simulink model "mainSIM"  (R2016a)
settings: Solver=VariableStepAuto  StartTime=0.0  StopTime=15  RelTol=1e-5
settings Model: Creator=Zoltan  LastModifiedBy=Zoltan

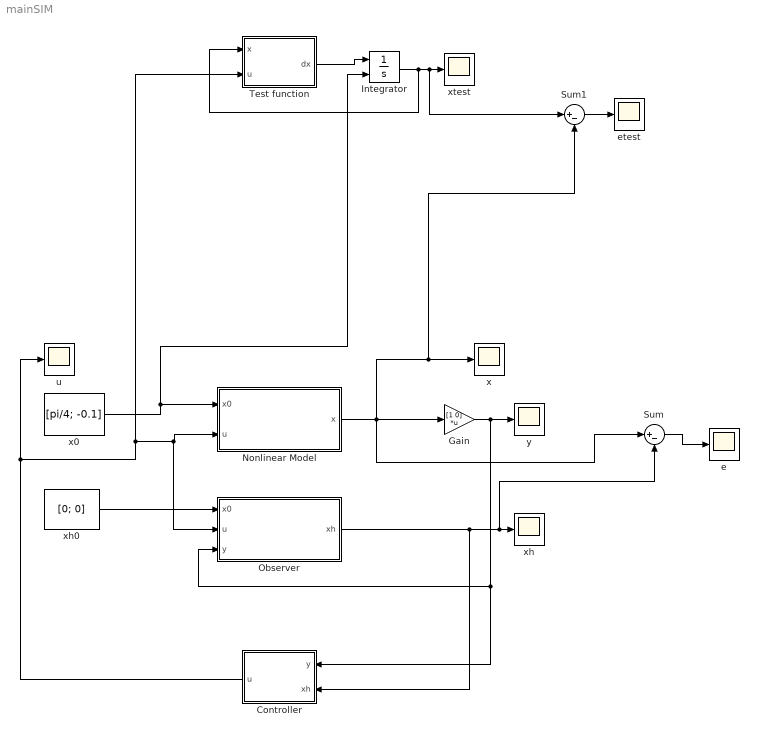
== system mainSIM ==
  Controller : MATLAB Function  TreatAsAtomicUnit=on
  Gain : Gain  Gain=[1 0]  Multiplication=Matrix(K*u) (u vector)
  Integrator : Integrator  InitialConditionSource=external
  Nonlinear Model : Subsystem
  Observer : Subsystem
  Sum : Sum  Inputs=|+-
  Sum1 : Sum  Inputs=|+-
  Test function : MATLAB Function  TreatAsAtomicUnit=on
  e : Scope
  etest : Scope
  "u " : Scope
  x : Scope
  x0 : Constant  Value=[pi/4; -0.1]
  xh : Scope
  xh0 : Constant  Value=[0; 0]
  xtest : Scope
  y : Scope
  wires:
  x0/1 -> Integrator/2, Nonlinear Model/1(x0)
  Controller/1(u) -> Test function/2(u), Observer/2(u), Nonlinear Model/2(u), "u "/1
  Nonlinear Model/1(x) -> Sum1/2, x/1, Sum/1, Gain/1
  Gain/1 -> Controller/1(y), Observer/3(y), y/1
  xh0/1 -> Observer/1(x0)
  Observer/1(xh) -> Controller/2(xh), Sum/2, xh/1
  Sum/1 -> e/1
  Test function/1(dx) -> Integrator/1
  Integrator/1 -> Test function/1(x), Sum1/1, xtest/1
  Sum1/1 -> etest/1

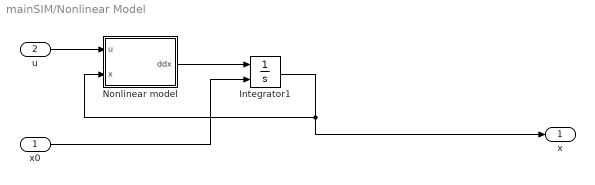
== system mainSIM/Nonlinear Model ==
  x0 : Inport
  u : Inport  Port=2
  Integrator1 : Integrator  InitialConditionSource=external
  Nonlinear model : MATLAB Function  TreatAsAtomicUnit=on
  x : Outport
  wires:
  u/1 -> Nonlinear model/1(u)
  x0/1 -> Integrator1/2
  Nonlinear model/1(ddx) -> Integrator1/1
  Integrator1/1 -> x/1, Nonlinear model/2(x)

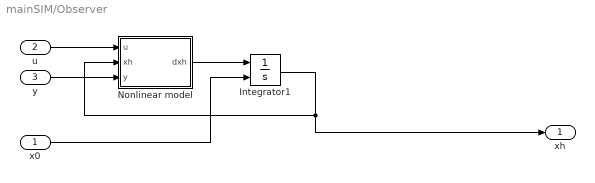
== system mainSIM/Observer ==
  x0 : Inport
  u : Inport  Port=2
  y : Inport  Port=3
  Integrator1 : Integrator  InitialConditionSource=external
  Nonlinear model : MATLAB Function  TreatAsAtomicUnit=on
  xh : Outport
  wires:
  u/1 -> Nonlinear model/1(u)
  x0/1 -> Integrator1/2
  Nonlinear model/1(dxh) -> Integrator1/1
  Integrator1/1 -> xh/1, Nonlinear model/2(xh)
  y/1 -> Nonlinear model/3(y)

== matlab function mainSIM/Observer/Nonlinear model ==
  data: u input; dxh output; xh input; y input
function dxh = fcn(u,xh,y)
coder.extrinsic('mydxh');
dxh= [0;0];
dxh = mydxh(y,xh,u);
y = u;

== matlab function mainSIM/Nonlinear Model/Nonlinear model ==
  data: u input; ddx output; x input
function ddx = fcn(u,x)
coder.extrinsic('mydx');
ddx= [0;0];
ddx = mydx(x,u);
y = u;

== matlab function mainSIM/Controller ==
  data: y input; xh input; u output
function u = fcn(y, xh)
coder.extrinsic('mycont');
u = 0;
u = mycont(y,xh);
%u = -u;
y = u;

== matlab function mainSIM/Test function ==
  data: x input; u input; dx output
function dx = fcn(x,u)
%#codegen
 g = 9.8;
 m = 0.3;
 M = 15;
 d = 0.007;
 l = 0.3;
 J = 0.005;
 a = 1/( M+ m);
% simulation params
sigm = 4;               % radian/s
x1 = x(1);
x2 = x(2);

alpha = ( J+ m* l^2)- a* m^2* l^2*cos(x1)^2;
rho1 = (- d+2*sigm* a* m* l*cos(x1)*sin(x1))/alpha;
rho2 = (- a* m* l*cos(x1))./alpha;
rho3 =  m* l*sin(x1);
psi = x2^2 + 2*sigm*x2;
dx = [x2; rho1*x2+rho2*rho3*psi+rho2*u];

end
